simulink model "nfo"  (R2023b)
settings: Solver=FixedStepAuto  StartTime=0.0  StopTime=10.0  FixedStep=1e-4  RelTol=1e-3
values from neighbouring files (symbols this model uses):
  flux = 0.0059    [nfo.sldd]
  if_init = 40.0    [nfo.sldd]
  L = 8.5E-5    [nfo.sldd]
  Pn = 5.0    [nfo.sldd]
  Rs = 0.035    [nfo.sldd]
  Ts = 0.0001    [nfo.sldd]
  Udc = 24.0    [nfo.sldd]
undefined symbols (not defined in the file or in its folder): DiscIntNeverNeededParam, magnitude, PLL_I, PLL_P, sigbuilder_block
libraries: slpidlib x4, dspstat3 x1, mcbplantlib x1, autolibpmsmexterior x1
(part 1 of 2)
settings Model: DataDictionary=nfo.sldd  Creator=Administrator  LastModifiedBy=yanke
settings OptimizationCC: DefaultParameterBehavior=Inlined  UseDivisionForNetSlopeComputation=on  GainParamInheritBuiltInType=on  UseFloatMulNetSlope=on  InlineInvariantSignals=on  PassReuseOutputArgsAs=Individual arguments  ZeroExternalMemoryAtStartup=off  ZeroInternalMemoryAtStartup=off  NoFixptDivByZeroProtection=on  EfficientFloat2IntCast=on  LifeSpan=1  OptimizeBlockOrder=speed  DifferentSizesBufferReuse=on  EfficientTunableParamExpr=on
settings DebuggingCC: ParameterTunabilityLossMsg=error  UnconnectedInputMsg=warning  UnconnectedOutputMsg=warning  UnconnectedLineMsg=warning
settings HardwareCC: ProdBitPerPointer=32  ProdBitPerSizeT=32  ProdBitPerPtrDiffT=32  ProdLargestAtomicInteger=Long  ProdLargestAtomicFloat=Double  ProdWordSize=32  ProdLongLongMode=on  ProdHWDeviceType=ARM Compatible->ARM Cortex-M
settings ModelReferenceCC: EnableRefExpFcnMdlSchedulingChecks=on
settings SFSimCC: MATLABDynamicMemAlloc=off
settings RTWCC: Description=Embedded Coder  SystemTargetFile=ert.tlc  GenCodeOnly=on  TemplateMakefile=ert_default_tmf  GenerateReport=on  LaunchReport=on  GenerateCodeReplacementReport=on  DLArmComputeVersion=19.05
settings CodeAppCC: ForceParamTrailComments=on  IgnoreCustomStorageClasses=off  OperatorAnnotations=on  SimulinkDataObjDesc=on  SFDataObjDesc=on  CustomSymbolStrGlobalVar=rt$N$M  CustomSymbolStrType=$N$M  CustomSymbolStrFcn=$N$M$F  CustomSymbolStrMacro=$N$M  InsertBlockDesc=on
settings ERTTargetCC: TargetLangStandard=C99 (ISO)  CodeReplacementLibrary=ARM Cortex-M  GenerateSampleERTMain=on  IncludeMdlTerminateFcn=off  CombineSignalStateStructs=on  SupportComplex=off  SupportNonInlinedSFcns=on  InlinedParameterPlacement=NonHierarchical  ERTCustomFileTemplate=example_file_process.tlc  ERTFilePackagingFormat=CompactWithDataFile

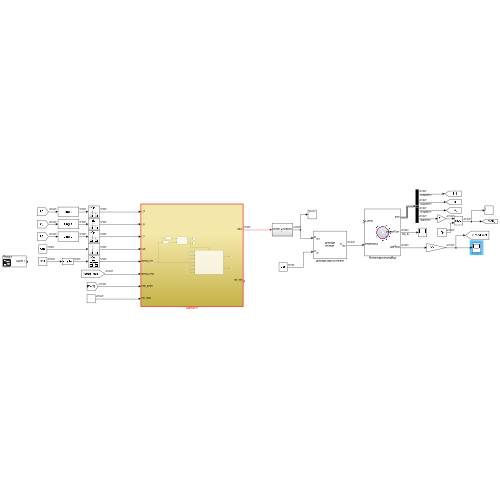
[thumbnail: Simulink's stored preview of the top-level diagram]
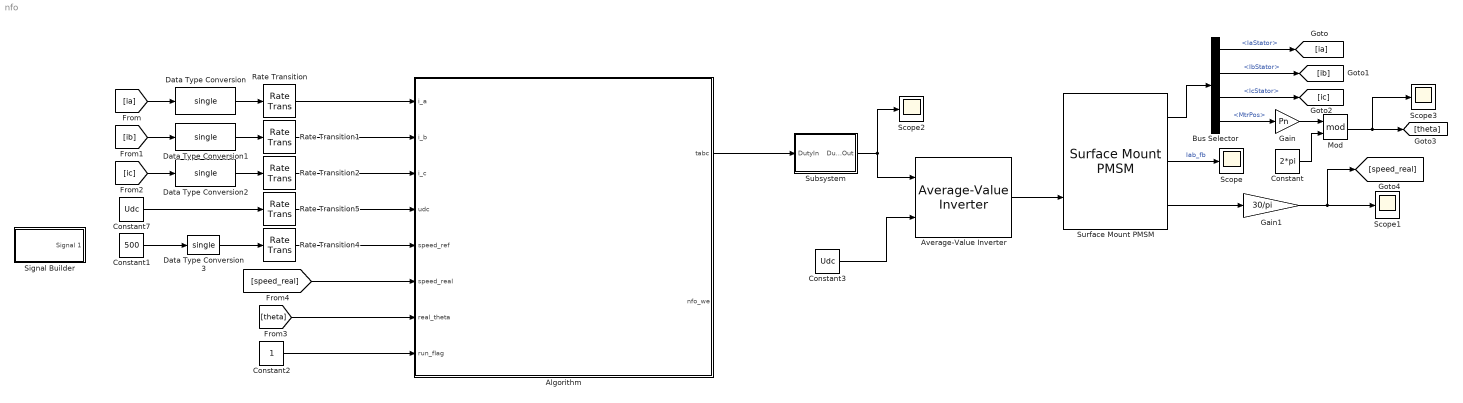
== system nfo ==
  Algorithm : Subsystem  TreatAsAtomicUnit=on
  Average-Value Inverter : mcbplantlib/Average-Value Inverter
  Bus Selector : BusSelector  OutputSignals=IaStator,IbStator,IcStator,MtrPos
  Constant : Constant  Value=2*pi
  Constant1 : Constant  Value=500
  Constant2 : Constant
  Constant3 : Constant  Value=Udc
  Constant7 : Constant  Value=Udc
  Data Type Conversion{,1..3} (4 alike) : DataTypeConversion  OutDataTypeStr=single  SaturateOnIntegerOverflow=off  RndMeth=Floor
  Gain : Gain  Gain=Pn
  Gain1 : Gain  Gain=30/pi
  Mod : Math  Operator=mod
  Rate Transition{,1..2,4..5} (5 alike) : RateTransition
  Scope{,1..3} (4 alike) : Scope
  Signal Builder : Subsystem  Tag=STV Subsys  LoadFcn=sigbuilder_block('load');  StartFcn=sigbuilder_block('start');  StopFcn=sigbuilder_block('stop');  ClipboardFcn=sigbuilder_block('clipboard');  mask(Sigbuilder block){tuvar=[0:10]}
      mask help: Simulink:masks:SigbuilderBlock_MD
      mask init:
      | if ~strcmp(get_param(bdroot(gcbh),'SimulationStatus'),'stopped') tuvar = sigbuilder_block('maskInit'); end
      settings: CopyFcn=sigbuilder_block('copy');  DeleteFcn=sigbuilder_block('delete');  ModelCloseFcn=sigbuilder_block('modelClose');  PreSaveFcn=sigbuilder_block('preSave');  PauseFcn=sigbuilder_block('pause');  ContinueFcn=sigbuilder_block('continue');  NameChangeFcn=sigbuilder_block('namechange');  OpenFcn=sigbuilder_block('open',[66 30 1269 684 ]);  CloseFcn=sigbuilder_block('close');
      mask Display: plot(0, 0, 100, 100,[2, 2, 32, 32, 2], [68, 8, 8, 68, 68],[32, 2], [38, 38], [32, 19, 2],[53, 60, 44], [32, 17, 17, 2],[16, 16, 31, 31]);txt = getActiveGroup(gcbh);text(2, 100, txt,'verticalAlignment', 'top');
  Subsystem : Subsystem
  Surface Mount PMSM : autolibpmsmexterior/Surface Mount PMSM  port_config=Torque  sim_type=Discrete  Ts=1e-4  P=Pn  Rs=Rs  Ldq_=L  KConstText=Permanent flux linkage constant (lambda_pm):  lambda_pm=flux  Ke=0.0059268  Kt=0.061  mechanical=[5.8e-5,0.0004924, 0]  idq0=[0 0]  theta_init=4/5  omega_init=0  KConst=flux  lambda_pm_calc=flux  RefBlkName='autolibpmsmexterior/Surface Mount PMSM'  aMode=5  Ldq="[0.0017      0.0017]"
  wires:
  Constant3/1 -> Average-Value Inverter/2
  Average-Value Inverter/1 -> Surface Mount PMSM/2
  Surface Mount PMSM/2 -> Scope/1  "Iab_fb"
  Surface Mount PMSM/1 -> Bus Selector/1
  Bus Selector/1 -> [ia]  "<IaStator>"
  Bus Selector/2 -> [ib]  "<IbStator>"
  Bus Selector/3 -> [ic]  "<IcStator>"
  Bus Selector/4 -> Gain/1  "<MtrPos>"
  Gain/1 -> Mod/1
  Constant/1 -> Mod/2
  Mod/1 -> Scope3/1, [theta]
  Data Type Conversion/1 -> Rate Transition/1
  [ia] -> Data Type Conversion/1
  [ib] -> Data Type Conversion1/1
  Data Type Conversion1/1 -> Rate Transition1/1
  Data Type Conversion2/1 -> Rate Transition2/1
  [ic] -> Data Type Conversion2/1
  Surface Mount PMSM/3 -> Gain1/1
  Gain1/1 -> [speed_real], Scope1/1
  Data Type Conversion3/1 -> Rate Transition4/1
  Subsystem/1(DutyOut) -> Average-Value Inverter/1, Scope2/1
  Algorithm/1(tabc) -> Subsystem/1(DutyIn)
  Rate Transition/1 -> Algorithm/1(i_a)
  Rate Transition1/1 -> Algorithm/2(i_b)
  Rate Transition2/1 -> Algorithm/3(i_c)
  Rate Transition5/1 -> Algorithm/4(udc)
  Constant7/1 -> Rate Transition5/1
  Rate Transition4/1 -> Algorithm/5(speed_ref)
  [speed_real] -> Algorithm/6(speed_real)
  [theta] -> Algorithm/7(real_theta)
  Constant2/1 -> Algorithm/8(run_flag)
  Constant1/1 -> Data Type Conversion3/1

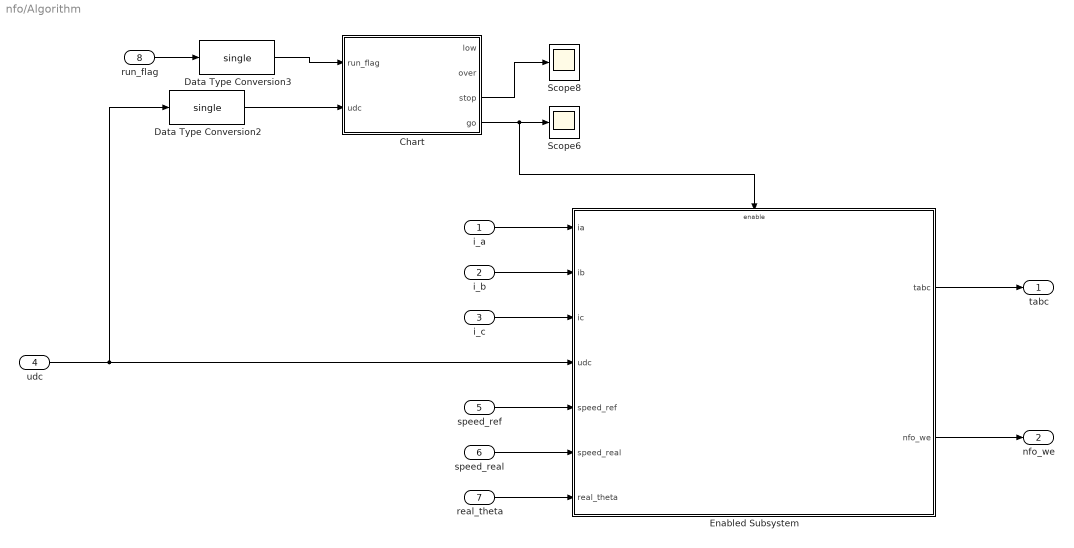
== system nfo/Algorithm ==
  i_a : Inport
  i_b : Inport  Port=2
  i_c : Inport  Port=3
  udc : Inport  Port=4
  speed_ref : Inport  Port=5
  speed_real : Inport  Port=6
  real_theta : Inport  Port=7
  run_flag : Inport  Port=8
  Chart : Stateflow chart  TreatAsAtomicUnit=on
  Data Type Conversion2 : DataTypeConversion  OutDataTypeStr=single  SaturateOnIntegerOverflow=off  RndMeth=Floor
  Data Type Conversion3 : DataTypeConversion  OutDataTypeStr=single  SaturateOnIntegerOverflow=off  RndMeth=Floor
  Enabled Subsystem : Subsystem  TreatAsAtomicUnit=on
  Scope6 : Scope
  Scope8 : Scope
  tabc : Outport
  nfo_we : Outport  Port=2
  wires:
  udc/1 -> Data Type Conversion2/1, Enabled Subsystem/4(udc)
  Data Type Conversion2/1 -> Chart/2(udc)
  run_flag/1 -> Data Type Conversion3/1
  Data Type Conversion3/1 -> Chart/1(run_flag)
  Chart/4(go) -> Enabled Subsystem/Enable, Scope6/1
  Chart/3(stop) -> Scope8/1
  i_a/1 -> Enabled Subsystem/1(ia)
  i_b/1 -> Enabled Subsystem/2(ib)
  i_c/1 -> Enabled Subsystem/3(ic)
  speed_ref/1 -> Enabled Subsystem/5(speed_ref)
  speed_real/1 -> Enabled Subsystem/6(speed_real)
  real_theta/1 -> Enabled Subsystem/7(real_theta)
  Enabled Subsystem/1(tabc) -> tabc/1
  Enabled Subsystem/2(nfo_we) -> nfo_we/1

== system nfo/Signal Builder ==
  Demux : Demux  Tag=STV Demux  Outputs=1
      settings: DisplayOption=none
  FromWs : FromWorkspace  Tag=STV FromWs  VariableName=tuvar
      SigBuilderData=|
      | common.afterFinalStr = 'Extrapolate'
      | common.sampleTime = 0
      | dataSet.timeRange = [0 10]
      | dataSet.name = 'Group 1'
      | sbobj.Groups.Name = 'Group 1'
      | sbobj.Groups.Signals.Name = 'Signal 1'
      | sbobj.Groups.Signals.XData = [0 4 4 7 7 10]
      | sbobj.Groups.Signals.YData = [302 302 700 700 -238 -238]
  Signal 1 : Outport  Tag=STV Outport
  wires:
  Demux/1 -> Signal 1/1
  FromWs/1 -> Demux/1

== system nfo/Subsystem ==
  DutyIn : Inport
  Constant : Constant  Value=0.5  SampleTime=-1
  Gain : Gain  Gain=1/8000  ParamDataTypeStr=single
  Gain1 : Gain  Gain=-1
  Sum : Sum  Inputs=|+-
  Sum1 : Sum  Inputs=|++
  DutyOut : Outport
  wires:
  Sum/1 -> Gain1/1
  Constant/1 -> Sum1/2, Sum/2
  DutyIn/1 -> Gain/1
  Gain1/1 -> Sum1/1
  Sum1/1 -> DutyOut/1
  Gain/1 -> Sum/1

== system nfo/Algorithm/Chart/low_vbus ==
  Input : Inport  OutDataTypeStr=single  PortDimensions=1
  f : TriggerPort  TriggerType=function-call  VariantControl=(inherit)
      settings: CopyFcn=Stateflow.SLINSF.SimulinkMan.removeBlockPreDeleteFcn  PreDeleteFcn=Stateflow.SLINSF.SimulinkMan.unsafePredeleteFcn
  Data Type Conversion : DataTypeConversion  OutDataTypeStr=boolean  SaturateOnIntegerOverflow=off  RndMeth=Floor
  Data Type Conversion1 : DataTypeConversion  OutDataTypeStr=single  SaturateOnIntegerOverflow=off  RndMeth=Floor
  NOR : Logic  Operator=NOT  IconShape=distinctive  OutDataTypeStr=boolean
  Relay : Relay  OnSwitchValue=20  OffSwitchValue=18
  out : Outport
  wires:
  Input/1 -> Relay/1
  Relay/1 -> Data Type Conversion/1
  Data Type Conversion/1 -> NOR/1
  NOR/1 -> Data Type Conversion1/1
  Data Type Conversion1/1 -> out/1

== system nfo/Algorithm/Chart/over_vbus ==
  Input : Inport  OutDataTypeStr=single  PortDimensions=1
  f : TriggerPort  TriggerType=function-call  VariantControl=(inherit)
      settings: CopyFcn=Stateflow.SLINSF.SimulinkMan.removeBlockPreDeleteFcn  PreDeleteFcn=Stateflow.SLINSF.SimulinkMan.unsafePredeleteFcn
  Relay : Relay  OnSwitchValue=28  OffSwitchValue=25
  out : Outport
  wires:
  Input/1 -> Relay/1
  Relay/1 -> out/1

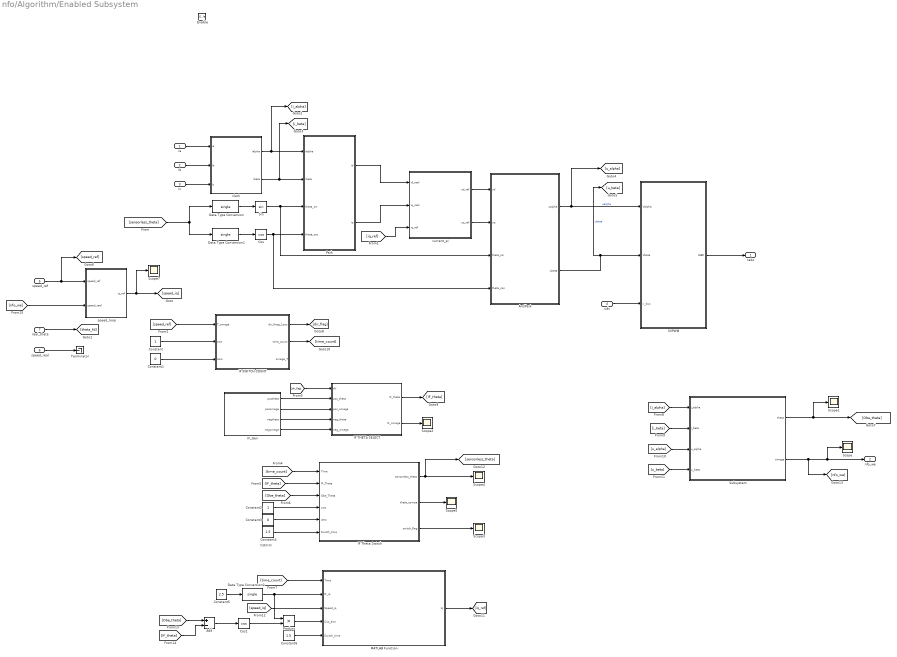
== system nfo/Algorithm/Enabled Subsystem ==
  note: 切换时间
  ia : Inport
  ib : Inport  Port=2
  ic : Inport  Port=3
  udc : Inport  Port=4
  speed_ref : Inport  Port=5
  speed_real : Inport  Port=6
  real_theta : Inport  Port=7
  Enable : EnablePort
  Add : Sum  Inputs=+-
  AntiPark : Subsystem
  Constant : Constant
  Constant1 : Constant  Value=0
  Constant2 : Constant  OutDataTypeStr=single
  Constant3 : Constant  Value=0  OutDataTypeStr=single
  Constant4 : Constant  Value=1.5  OutDataTypeStr=single
  Constant5 : Constant  Value=2.5
  Constant6 : Constant  Value=1.5
  Cos : Trigonometry  Operator=cos
  Cos1 : Trigonometry  Operator=cos
  Data Type Conversion : DataTypeConversion  OutDataTypeStr=single  SaturateOnIntegerOverflow=off  RndMeth=Floor
  Data Type Conversion1 : DataTypeConversion  OutDataTypeStr=single  SaturateOnIntegerOverflow=off  RndMeth=Floor
  Data Type Conversion2 : DataTypeConversion  OutDataTypeStr=single  SaturateOnIntegerOverflow=off  RndMeth=Floor
  IF SWITCH COUNT : MATLAB Function  TreatAsAtomicUnit=on
  IF THETA SELECT : MATLAB Function  TreatAsAtomicUnit=on
  "IF Theta Switch " : MATLAB Function  TreatAsAtomicUnit=on
  IF_Gen : Subsystem
  MATLAB Function : MATLAB Function  TreatAsAtomicUnit=on
  Park : Subsystem
  Product : Product
  SVPWM : Subsystem  TreatAsAtomicUnit=on
  Scope{,1..5,7} (7 alike) : Scope
  Sin : Trigonometry
  Subsystem : Subsystem
  Terminator : Terminator
  clark : Subsystem
  current_pi : Subsystem
  speed_loop : Subsystem
  tabc : Outport  OutputWhenDisabled=reset  InitialOutput=0
  nfo_we : Outport  Port=2
  wires:
  ic/1 -> clark/3(ic)
  AntiPark/2(ubeta) -> SVPWM/2(Vbeta), [u_beta]  "ubeta"
  IF_Gen/2(posomega) -> IF THETA SELECT/3(pos_omega)
  Data Type Conversion/1 -> Sin/1
  Park/1(id) -> current_pi/1(id_real)
  IF THETA SELECT/2(IF_omega) -> Scope2/1
  [i_alpha] -> Subsystem/1(i_alpha)
  ib/1 -> clark/2(ib)
  [speed_iq] -> MATLAB Function/3(Speed_iq)
  IF_Gen/1(postheta) -> IF THETA SELECT/2(pos_theta)
  Cos/1 -> AntiPark/4(theta_cos), Park/4(theta_cos)
  AntiPark/1(ualpha) -> [u_alpha], SVPWM/1(Valpha)  "ualpha"
  [time_count] -> MATLAB Function/1(Time)
  Subsystem/2(omega) -> [nfo_we], Scope/1, nfo_we/1
  Constant3/1 -> "IF Theta Switch "/5(zero)
  Sin/1 -> AntiPark/3(theta_sin), Park/3(theta_sin)
  IF SWITCH COUNT/1(dir_0neg_1pos) -> [dir_flag]
  "IF Theta Switch "/2(theta_compa) -> Scope5/1
  [i_beta] -> Subsystem/2(i_beta)
  Data Type Conversion1/1 -> Cos/1
  Constant6/1 -> MATLAB Function/5(Switch_time)
  Cos1/1 -> Product/2
  udc/1 -> SVPWM/3(v_bus)
  [sensorless_theta] -> Data Type Conversion/1, Data Type Conversion1/1
  [Obe_theta] -> Add/1
  [u_beta] -> Subsystem/4(u_beta)
  [iq_ref] -> current_pi/3(iq_ref)
  speed_ref/1 -> [speed_ref], speed_loop/1(speed_ref)
  clark/1(ialpha) -> [i_alpha], Park/1(ialpha)
  [u_alpha] -> Subsystem/3(u_alpha)
  IF_Gen/4(negomega) -> IF THETA SELECT/5(neg_omega)
  Subsystem/1(theta) -> Scope1/1, [Obe_theta]
  SVPWM/1(tABC) -> tabc/1
  ia/1 -> clark/1(ia)
  "IF Theta Switch "/1(sensorless_theta) -> Scope4/1, [sensorless_theta]
  real_theta/1 -> [theta_fd]
  [speed_ref] -> IF SWITCH COUNT/1(T_omega)
  Constant/1 -> IF SWITCH COUNT/2(one)
  [dir_flag] -> IF THETA SELECT/1(dir)
  current_pi/2(uq_ref) -> AntiPark/2(uq)
  Constant1/1 -> IF SWITCH COUNT/3(zero)
  clark/2(ibeta) -> [i_beta], Park/2(ibeta)
  [time_count] -> "IF Theta Switch "/1(Time)
  [Obe_theta] -> "IF Theta Switch "/3(Obe_Theta)
  Constant2/1 -> "IF Theta Switch "/4(one)
  [IF_theta] -> "IF Theta Switch "/2(IF_Theta)
  Park/2(iq) -> current_pi/2(iq_real)
  "IF Theta Switch "/3(switch_flag) -> Scope3/1
  Constant5/1 -> Data Type Conversion2/1
  IF THETA SELECT/1(IF_theta) -> [IF_theta]
  IF SWITCH COUNT/2(time_count) -> [time_count]
  IF_Gen/3(negtheta) -> IF THETA SELECT/4(neg_theta)
  Product/1 -> MATLAB Function/4(Cos_eror)
  Add/1 -> Cos1/1
  Constant4/1 -> "IF Theta Switch "/6(Switch_time)
  current_pi/1(ud_ref) -> AntiPark/1(ud)
  speed_loop/1(iq_ref) -> Scope7/1, [speed_iq]
  [IF_theta] -> Add/2
  MATLAB Function/1(Iq) -> [iq_ref]
  speed_real/1 -> Terminator/1
  [nfo_we] -> speed_loop/2(speed_real)
  Data Type Conversion2/1 -> Product/1, MATLAB Function/2(IF_iq)

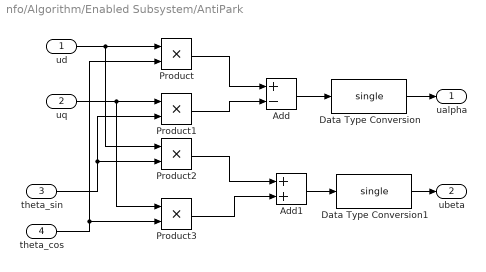
== system nfo/Algorithm/Enabled Subsystem/AntiPark ==
  ud : Inport
  uq : Inport  Port=2
  theta_sin : Inport  Port=3
  theta_cos : Inport  Port=4
  Add : Sum  Inputs=+-
  Add1 : Sum
  Data Type Conversion : DataTypeConversion  OutDataTypeStr=single  SaturateOnIntegerOverflow=off  RndMeth=Floor
  Data Type Conversion1 : DataTypeConversion  OutDataTypeStr=single  SaturateOnIntegerOverflow=off  RndMeth=Floor
  Product{,1..3} (4 alike) : Product
  ualpha : Outport  OutDataTypeStr=single
  ubeta : Outport  Port=2  OutDataTypeStr=single
  wires:
  Add1/1 -> Data Type Conversion1/1
  Product1/1 -> Add/2
  uq/1 -> Product3/1, Product1/1
  theta_cos/1 -> Product/2, Product3/2
  theta_sin/1 -> Product2/2, Product1/2
  ud/1 -> Product2/1, Product/1
  Product3/1 -> Add1/2
  Add/1 -> Data Type Conversion/1
  Product/1 -> Add/1
  Product2/1 -> Add1/1
  Data Type Conversion/1 -> ualpha/1
  Data Type Conversion1/1 -> ubeta/1

== system nfo/Algorithm/Enabled Subsystem/IF_Gen ==
  note: 对常数项积分，得到omega，在对omeg积分，得到theta
  IFneg : Subsystem  TreatAsAtomicUnit=on
      mask Display:
      | port_label('output',1,'negtheta','texmode','on');
      | port_label('output',2,'negomega','texmode','on');
      | 
      | fprintf('IFneg_theta');
  IFpos : Subsystem  TreatAsAtomicUnit=on
      mask Display:
      | port_label('output',1,'postheta','texmode','on');
      | port_label('output',2,'posomega','texmode','on');
      | 
      | fprintf('IFpos_theta');
  postheta : Outport
  posomega : Outport  Port=2
  negtheta : Outport  Port=3
  negomega : Outport  Port=4
  wires:
  IFpos/1(theta) -> postheta/1
  IFneg/2(omega) -> negomega/1
  IFneg/1(theta) -> negtheta/1
  IFpos/2(omega) -> posomega/1

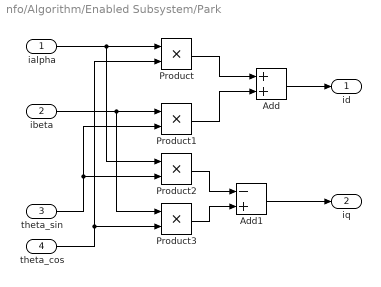
== system nfo/Algorithm/Enabled Subsystem/Park ==
  ialpha : Inport  OutDataTypeStr=single
  ibeta : Inport  Port=2  OutDataTypeStr=single
  theta_sin : Inport  Port=3  OutDataTypeStr=single
  theta_cos : Inport  Port=4  OutDataTypeStr=single
  Add : Sum  OutDataTypeStr=single  AccumDataTypeStr=single
  Add1 : Sum  Inputs=-+  OutDataTypeStr=single  AccumDataTypeStr=single
  Product{,1..3} (4 alike) : Product  OutDataTypeStr=single
  id : Outport  OutDataTypeStr=single
  iq : Outport  Port=2  OutDataTypeStr=single
  wires:
  theta_cos/1 -> Product/2, Product3/2
  ibeta/1 -> Product1/1, Product3/1
  Product1/1 -> Add/2
  Add1/1 -> iq/1
  Add/1 -> id/1
  Product3/1 -> Add1/2
  ialpha/1 -> Product/1, Product2/1
  Product2/1 -> Add1/1
  Product/1 -> Add/1
  theta_sin/1 -> Product1/2, Product2/2

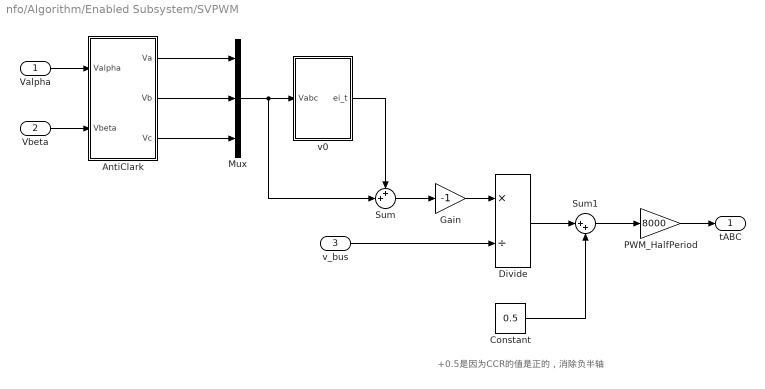
== system nfo/Algorithm/Enabled Subsystem/SVPWM ==
  note: +0.5是因为CCR的值是正的，消除负半轴
  Valpha : Inport  OutDataTypeStr=single
  Vbeta : Inport  Port=2  OutDataTypeStr=single
  v_bus : Inport  Port=3  OutDataTypeStr=single
  AntiClark : Subsystem
  Constant : Constant  Value=0.5  OutDataTypeStr=single
  Divide : Product  Inputs=*/  OutDataTypeStr=single
  Gain : Gain  Gain=-1  OutDataTypeStr=single
  Mux : Mux  Inputs=3
  PWM_HalfPeriod : Gain  Gain=8000  OutDataTypeStr=single
  Sum : Sum  Inputs=++|  OutDataTypeStr=single
  Sum1 : Sum  Inputs=|++  OutDataTypeStr=single
  v0 : Subsystem
  tABC : Outport  OutDataTypeStr=single
  wires:
  Valpha/1 -> AntiClark/1(Valpha)
  Vbeta/1 -> AntiClark/2(Vbeta)
  v0/1(ei_t) -> Sum/1
  AntiClark/1(Va) -> Mux/1
  AntiClark/2(Vb) -> Mux/2
  AntiClark/3(Vc) -> Mux/3
  Sum/1 -> Gain/1
  Mux/1 -> Sum/2, v0/1(Vabc)
  Divide/1 -> Sum1/1
  Constant/1 -> Sum1/2
  Sum1/1 -> PWM_HalfPeriod/1
  PWM_HalfPeriod/1 -> tABC/1
  v_bus/1 -> Divide/2
  Gain/1 -> Divide/1

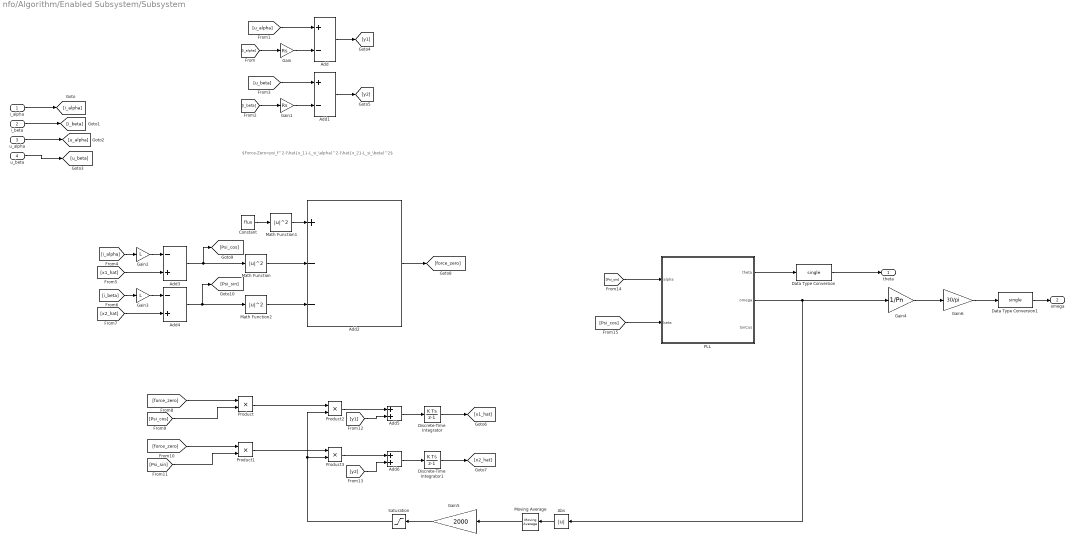
== system nfo/Algorithm/Enabled Subsystem/Subsystem ==
  note: $Force-Zero=psi_f^2-(\hat{x_1}-L_si_\alpha)^2-(\hat{x_2}-L_si_\beta)^2$
  i_alpha : Inport
  i_beta : Inport  Port=2
  u_alpha : Inport  Port=3
  u_beta : Inport  Port=4
  Abs : Abs  OutDataTypeStr=single  SaturateOnIntegerOverflow=off
  Add : Sum  Inputs=+-
  Add1 : Sum  Inputs=+-
  Add2 : Sum  Inputs=+--
  Add3 : Sum  Inputs=-+
  Add4 : Sum  Inputs=-+
  Add5 : Sum
  Add6 : Sum
  Constant : Constant  Value=flux
  Data Type Conversion : DataTypeConversion  OutDataTypeStr=single  SaturateOnIntegerOverflow=off  RndMeth=Floor
  Data Type Conversion1 : DataTypeConversion  OutDataTypeStr=single  SaturateOnIntegerOverflow=off  RndMeth=Floor
  Discrete-Time Integrator : DiscreteIntegrator  InitialCondition=0.011  SampleTime=-1  ICPrevOutput=DiscIntNeverNeededParam  ICPrevScaledInput=DiscIntNeverNeededParam
  Discrete-Time Integrator1 : DiscreteIntegrator  InitialCondition=-0.011  SampleTime=-1  ICPrevOutput=DiscIntNeverNeededParam  ICPrevScaledInput=DiscIntNeverNeededParam
  Gain : Gain  Gain=Rs
  Gain1 : Gain  Gain=Rs
  Gain2 : Gain  Gain=L
  Gain3 : Gain  Gain=L
  Gain4 : Gain  Gain=1/Pn
  Gain5 : Gain  Gain=2000  OutDataTypeStr=single
  Gain6 : Gain  Gain=30/pi
  Math Function : Math  Operator=magnitude^2
  Math Function1 : Math  Operator=magnitude^2
  Math Function2 : Math  Operator=magnitude^2
  Moving Average : dspstat3/Moving Average  Method=Exponential weighting  ForgettingFactorPort=off  SpecifyWindowLength=on  WindowLength=4  OverlapLength=3  AllowArbitraryInputLength=off  ForgettingFactor=0.99  SimulateUsing=Code generation
  PLL : Subsystem
  Product{,1..3} (4 alike) : Product
  Saturation : Saturate  UpperLimit=500e4  LowerLimit=100000  OutDataTypeStr=single
  theta : Outport
  omega : Outport  Port=2
  wires:
  i_alpha/1 -> [i_alpha]
  i_beta/1 -> [i_beta]
  [i_alpha] -> Gain/1
  Gain/1 -> Add/2
  u_alpha/1 -> [u_alpha]
  u_beta/1 -> [u_beta]
  [u_alpha] -> Add/1
  Gain1/1 -> Add1/2
  [i_beta] -> Gain1/1
  [u_beta] -> Add1/1
  Add/1 -> [y1]
  Add1/1 -> [y2]
  Constant/1 -> Math Function1/1
  [i_alpha] -> Gain2/1
  Gain2/1 -> Add3/1
  [x1_hat] -> Add3/2
  Add3/1 -> [Psi_cos], Math Function/1
  Math Function1/1 -> Add2/1
  Math Function/1 -> Add2/2
  [i_beta] -> Gain3/1
  [x2_hat] -> Add4/2
  Add4/1 -> [Psi_sin], Math Function2/1
  Gain3/1 -> Add4/1
  Math Function2/1 -> Add2/3
  Add2/1 -> [force_zero]
  [force_zero] -> Product/1
  [Psi_cos] -> Product/2
  [force_zero] -> Product1/1
  [Psi_sin] -> Product1/2
  Product1/1 -> Product3/1
  Product/1 -> Product2/1
  Product2/1 -> Add5/1
  [y1] -> Add5/2
  Product3/1 -> Add6/1
  [y2] -> Add6/2
  Add5/1 -> Discrete-Time Integrator/1
  Discrete-Time Integrator/1 -> [x1_hat]
  Add6/1 -> Discrete-Time Integrator1/1
  Discrete-Time Integrator1/1 -> [x2_hat]
  Abs/1 -> Moving Average/1
  Moving Average/1 -> Gain5/1
  Gain5/1 -> Saturation/1
  Saturation/1 -> Product2/2, Product3/2
  Gain4/1 -> Gain6/1
  Gain6/1 -> Data Type Conversion1/1
  Data Type Conversion1/1 -> omega/1
  Data Type Conversion/1 -> theta/1
  [Psi_sin] -> PLL/1(alpha)
  [Psi_cos] -> PLL/2(beta)
  PLL/1(theta) -> Data Type Conversion/1
  PLL/2(omega) -> Gain4/1, Abs/1

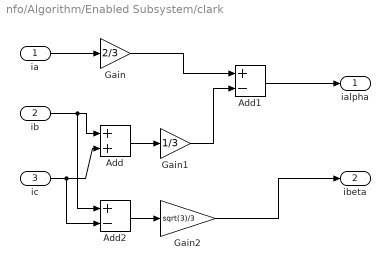
== system nfo/Algorithm/Enabled Subsystem/clark ==
  ia : Inport  OutDataTypeStr=single
  ib : Inport  Port=2  OutDataTypeStr=single
  ic : Inport  Port=3  OutDataTypeStr=single
  Add : Sum  OutDataTypeStr=single  AccumDataTypeStr=single
  Add1 : Sum  Inputs=+-  OutDataTypeStr=single  AccumDataTypeStr=single
  Add2 : Sum  Inputs=+-  OutDataTypeStr=single  AccumDataTypeStr=single
  Gain : Gain  Gain=2/3  ParamDataTypeStr=single
  Gain1 : Gain  Gain=1/3  ParamDataTypeStr=single
  Gain2 : Gain  Gain=sqrt(3)/3  ParamDataTypeStr=single
  ialpha : Outport  OutDataTypeStr=single
  ibeta : Outport  Port=2  OutDataTypeStr=single
  wires:
  ib/1 -> Add/1, Add2/1
  Gain1/1 -> Add1/2
  Add2/1 -> Gain2/1
  Add1/1 -> ialpha/1
  Gain/1 -> Add1/1
  ic/1 -> Add/2, Add2/2
  ia/1 -> Gain/1
  Add/1 -> Gain1/1
  Gain2/1 -> ibeta/1

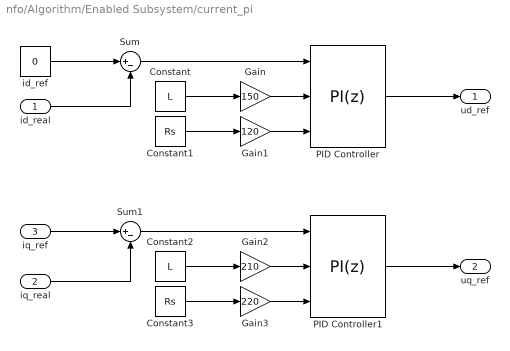
== system nfo/Algorithm/Enabled Subsystem/current_pi ==
  id_real : Inport
  iq_real : Inport  Port=2
  iq_ref : Inport  Port=3
  Constant : Constant  Value=L
  Constant1 : Constant  Value=Rs
  Constant2 : Constant  Value=L
  Constant3 : Constant  Value=Rs
  Gain : Gain  Gain=150
  Gain1 : Gain  Gain=120
  Gain2 : Gain  Gain=210
  Gain3 : Gain  Gain=220
  PID Controller : slpidlib/PID Controller  Controller=PI  Form=Parallel  TimeDomain=Discrete-time  UseExternalTs=off  SampleTime=-1  IntegratorMethod=Forward Euler  FilterMethod=Forward Euler  ControllerParametersSource=external  P=1  I=1  UseKiTs=off  D=0  N=100  UseFilter=on  TunerSelectOption=Transfer Function Based (PID Tuner App)  InitialConditionSource=internal  InitialConditionForIntegrator=0  InitialConditionForFilter=0  DifferentiatorICPrevScaledInput=0  ExternalReset=none  TrackingMode=off  Kt=1  LimitOutput=on  SatLimitsSource=internal  UpperSaturationLimit=Udc*0.9/sqrt(3)  LowerSaturationLimit=-Udc*0.9/sqrt(3)  LinearizeAsGain=on  AntiWindupMode=clamping  Kb=1  LimitIntegrator=off  UpperIntegratorSaturationLimit=inf  LowerIntegratorSaturationLimit=-inf  POutMin=[]  POutMax=[]  IOutMin=[]  IOutMax=[]  DOutMin=[]  DOutMax=[]  NOutMin=[]  NOutMax=[]  SumOutMin=[]  SumOutMax=[]  SaturationOutMin=[]  SaturationOutMax=[]  PParamMin=[]  PParamMax=[]  IParamMin=[]  IParamMax=[]  DParamMin=[]  DParamMax=[]  NParamMin=[]  NParamMax=[]  KbParamMin=[]  KbParamMax=[]  KtParamMin=[]  KtParamMax=[]  KbOutMin=[]  KbOutMax=[]  KtOutMin=[]  KtOutMax=[]  IntegratorOutMin=[]  IntegratorOutMax=[]  FilterOutMin=[]  FilterOutMax=[]  SumI1OutMin=[]  SumI1OutMax=[]  SumI2OutMin=[]  SumI2OutMax=[]  SumI3OutMin=[]  SumI3OutMax=[]  SumI4OutMin=[]  SumI4OutMax=[]  SumDOutMin=[]  SumDOutMax=[]  DifferentiatorOutMin=[]  DifferentiatorOutMax=[]  FilterDiffOutCoefMin=[]  FilterDiffOutCoefMax=[]  ReciprocalOutMin=[]  ReciprocalOutMax=[]  SumDenOutMin=[]  SumDenOutMax=[]  SumNumOutMin=[]  SumNumOutMax=[]  DivideOutMin=[]  DivideOutMax=[]  UdiffTsProdOutMin=[]  UdiffTsProdOutMax=[]  NTsProdOutMin=[]  NTsProdOutMax=[]  UintegralTsProdOutMin=[]  UintegralTsProdOutMax=[]  UngainTsProdOutMin=[]  UngainTsProdOutMax=[]  ClampingZeroOutDataTypeStr=Inherit: Inherit via back propagation  ClampingZeroOutMin=[]  ClampingZeroOutMax=[]  FilterDenConstantOutDataTypeStr=Inherit: Inherit via back propagation  FilterDenConstantOutMin=[]  FilterDenConstantOutMax=[]  PCopyOutDataTypeStr=Inherit: Inherit via back propagation  PCopyOutMin=[]  PCopyOutMax=[]  NCopyOutDataTypeStr=Inherit: Inherit via back propagation  NCopyOutMin=[]  NCopyOutMax=[]  IntegratorContinuousStateAttributes=''  IntegratorStateMustResolveToSignalObject=off  IntegratorRTWStateStorageClass=Auto  FilterContinuousStateAttributes=''  FilterStateMustResolveToSignalObject=off  FilterRTWStateStorageClass=Auto  ParallelPVariant=ExternalParameters  IdealPVariant=Disabled  IVariant=ExternalParameters  DVariant=Disabled  IntegratorVariant=Discrete  SatVariant=Enabled  AWVariant=DiscClampingParallel  PCopyVariant=Disabled  TRVariant=Disabled  FdbkBlocksVariant=Forward  IdealPFdbkVariant=Disabled  SatFdbkVariant=Disabled  DerivativeFilterVariant=Disabled  NVariant=Disabled  NCopyVariant=Disabled_SignalSpec  FilterICVariant=Disabled  IntegratorICVariant=InternalICs  ExternalResetVariant=Disabled  TRSumVariant=Passthrough  SumFdbkVariant=Disabled  SumVariant=Sum_PI  TsampFilterVariant=InternalTs  TsampNgainVariant=Passthrough  TsampIntegralVariant=Disabled_SignalSpec  ExternalSaturationOutDataTypeStr=Inherit: Same as second input
  PID Controller1 : slpidlib/PID Controller  Controller=PI  Form=Parallel  TimeDomain=Discrete-time  UseExternalTs=off  SampleTime=-1  IntegratorMethod=Forward Euler  FilterMethod=Forward Euler  ControllerParametersSource=external  P=1  I=1  UseKiTs=off  D=0  N=100  UseFilter=on  TunerSelectOption=Transfer Function Based (PID Tuner App)  InitialConditionSource=internal  InitialConditionForIntegrator=0  InitialConditionForFilter=0  DifferentiatorICPrevScaledInput=0  ExternalReset=none  TrackingMode=off  Kt=1  LimitOutput=on  SatLimitsSource=internal  UpperSaturationLimit=Udc*0.9/sqrt(3)  LowerSaturationLimit=-Udc*0.9/sqrt(3)  LinearizeAsGain=on  AntiWindupMode=clamping  Kb=1  LimitIntegrator=off  UpperIntegratorSaturationLimit=inf  LowerIntegratorSaturationLimit=-inf  POutMin=[]  POutMax=[]  IOutMin=[]  IOutMax=[]  DOutMin=[]  DOutMax=[]  NOutMin=[]  NOutMax=[]  SumOutMin=[]  SumOutMax=[]  SaturationOutMin=[]  SaturationOutMax=[]  PParamMin=[]  PParamMax=[]  IParamMin=[]  IParamMax=[]  DParamMin=[]  DParamMax=[]  NParamMin=[]  NParamMax=[]  KbParamMin=[]  KbParamMax=[]  KtParamMin=[]  KtParamMax=[]  KbOutMin=[]  KbOutMax=[]  KtOutMin=[]  KtOutMax=[]  IntegratorOutMin=[]  IntegratorOutMax=[]  FilterOutMin=[]  FilterOutMax=[]  SumI1OutMin=[]  SumI1OutMax=[]  SumI2OutMin=[]  SumI2OutMax=[]  SumI3OutMin=[]  SumI3OutMax=[]  SumI4OutMin=[]  SumI4OutMax=[]  SumDOutMin=[]  SumDOutMax=[]  DifferentiatorOutMin=[]  DifferentiatorOutMax=[]  FilterDiffOutCoefMin=[]  FilterDiffOutCoefMax=[]  ReciprocalOutMin=[]  ReciprocalOutMax=[]  SumDenOutMin=[]  SumDenOutMax=[]  SumNumOutMin=[]  SumNumOutMax=[]  DivideOutMin=[]  DivideOutMax=[]  UdiffTsProdOutMin=[]  UdiffTsProdOutMax=[]  NTsProdOutMin=[]  NTsProdOutMax=[]  UintegralTsProdOutMin=[]  UintegralTsProdOutMax=[]  UngainTsProdOutMin=[]  UngainTsProdOutMax=[]  ClampingZeroOutDataTypeStr=Inherit: Inherit via back propagation  ClampingZeroOutMin=[]  ClampingZeroOutMax=[]  FilterDenConstantOutDataTypeStr=Inherit: Inherit via back propagation  FilterDenConstantOutMin=[]  FilterDenConstantOutMax=[]  PCopyOutDataTypeStr=Inherit: Inherit via back propagation  PCopyOutMin=[]  PCopyOutMax=[]  NCopyOutDataTypeStr=Inherit: Inherit via back propagation  NCopyOutMin=[]  NCopyOutMax=[]  IntegratorContinuousStateAttributes=''  IntegratorStateMustResolveToSignalObject=off  IntegratorRTWStateStorageClass=Auto  FilterContinuousStateAttributes=''  FilterStateMustResolveToSignalObject=off  FilterRTWStateStorageClass=Auto  ParallelPVariant=ExternalParameters  IdealPVariant=Disabled  IVariant=ExternalParameters  DVariant=Disabled  IntegratorVariant=Discrete  SatVariant=Enabled  AWVariant=DiscClampingParallel  PCopyVariant=Disabled  TRVariant=Disabled  FdbkBlocksVariant=Forward  IdealPFdbkVariant=Disabled  SatFdbkVariant=Disabled  DerivativeFilterVariant=Disabled  NVariant=Disabled  NCopyVariant=Disabled_SignalSpec  FilterICVariant=Disabled  IntegratorICVariant=InternalICs  ExternalResetVariant=Disabled  TRSumVariant=Passthrough  SumFdbkVariant=Disabled  SumVariant=Sum_PI  TsampFilterVariant=InternalTs  TsampNgainVariant=Passthrough  TsampIntegralVariant=Disabled_SignalSpec  ExternalSaturationOutDataTypeStr=Inherit: Same as second input
  Sum : Sum  Inputs=|+-
  Sum1 : Sum  Inputs=|+-
  id_ref : Constant  Value=0
  ud_ref : Outport
  uq_ref : Outport  Port=2
  wires:
  id_ref/1 -> Sum/1
  id_real/1 -> Sum/2
  Sum/1 -> PID Controller/1
  PID Controller/1 -> ud_ref/1
  Gain/1 -> PID Controller/2
  Constant/1 -> Gain/1
  Gain1/1 -> PID Controller/3
  Constant1/1 -> Gain1/1
  Gain3/1 -> PID Controller1/3
  Constant2/1 -> Gain2/1
  Constant3/1 -> Gain3/1
  Gain2/1 -> PID Controller1/2
  Sum1/1 -> PID Controller1/1
  iq_ref/1 -> Sum1/1
  iq_real/1 -> Sum1/2
  PID Controller1/1 -> uq_ref/1

== system nfo/Algorithm/Enabled Subsystem/speed_loop ==
  note: 1.3 0.1
  speed_ref : Inport
  speed_real : Inport  Port=2
  PID Controller : slpidlib/PID Controller  Controller=PI  Form=Parallel  TimeDomain=Discrete-time  UseExternalTs=off  SampleTime=-1  IntegratorMethod=Forward Euler  FilterMethod=Forward Euler  ControllerParametersSource=internal  P=0.3  I=0.0003  UseKiTs=off  D=0  N=100  UseFilter=on  TunerSelectOption=Transfer Function Based (PID Tuner App)  InitialConditionSource=internal  InitialConditionForIntegrator=0  InitialConditionForFilter=0  DifferentiatorICPrevScaledInput=0  ExternalReset=none  TrackingMode=off  Kt=1  LimitOutput=on  SatLimitsSource=internal  UpperSaturationLimit=7  LowerSaturationLimit=-7  LinearizeAsGain=on  AntiWindupMode=clamping  Kb=1  LimitIntegrator=off  UpperIntegratorSaturationLimit=inf  LowerIntegratorSaturationLimit=-inf  POutMin=[]  POutMax=[]  IOutMin=[]  IOutMax=[]  DOutMin=[]  DOutMax=[]  NOutMin=[]  NOutMax=[]  SumOutMin=[]  SumOutMax=[]  SaturationOutMin=[]  SaturationOutMax=[]  PParamMin=[]  PParamMax=[]  IParamMin=[]  IParamMax=[]  DParamMin=[]  DParamMax=[]  NParamMin=[]  NParamMax=[]  KbParamMin=[]  KbParamMax=[]  KtParamMin=[]  KtParamMax=[]  KbOutMin=[]  KbOutMax=[]  KtOutMin=[]  KtOutMax=[]  IntegratorOutMin=[]  IntegratorOutMax=[]  FilterOutMin=[]  FilterOutMax=[]  SumI1OutMin=[]  SumI1OutMax=[]  SumI2OutMin=[]  SumI2OutMax=[]  SumI3OutMin=[]  SumI3OutMax=[]  SumI4OutMin=[]  SumI4OutMax=[]  SumDOutMin=[]  SumDOutMax=[]  DifferentiatorOutMin=[]  DifferentiatorOutMax=[]  FilterDiffOutCoefMin=[]  FilterDiffOutCoefMax=[]  ReciprocalOutMin=[]  ReciprocalOutMax=[]  SumDenOutMin=[]  SumDenOutMax=[]  SumNumOutMin=[]  SumNumOutMax=[]  DivideOutMin=[]  DivideOutMax=[]  UdiffTsProdOutMin=[]  UdiffTsProdOutMax=[]  NTsProdOutMin=[]  NTsProdOutMax=[]  UintegralTsProdOutMin=[]  UintegralTsProdOutMax=[]  UngainTsProdOutMin=[]  UngainTsProdOutMax=[]  ClampingZeroOutDataTypeStr=Inherit: Inherit via back propagation  ClampingZeroOutMin=[]  ClampingZeroOutMax=[]  FilterDenConstantOutDataTypeStr=Inherit: Inherit via back propagation  FilterDenConstantOutMin=[]  FilterDenConstantOutMax=[]  PCopyOutDataTypeStr=Inherit: Inherit via back propagation  PCopyOutMin=[]  PCopyOutMax=[]  NCopyOutDataTypeStr=Inherit: Inherit via back propagation  NCopyOutMin=[]  NCopyOutMax=[]  IntegratorContinuousStateAttributes=''  IntegratorStateMustResolveToSignalObject=off  IntegratorRTWStateStorageClass=Auto  FilterContinuousStateAttributes=''  FilterStateMustResolveToSignalObject=off  FilterRTWStateStorageClass=Auto  ParallelPVariant=InternalParameters  IdealPVariant=Disabled  IVariant=InternalParameters  DVariant=Disabled  IntegratorVariant=Discrete  SatVariant=Enabled  AWVariant=DiscClampingParallel  PCopyVariant=Disabled  TRVariant=Disabled  FdbkBlocksVariant=Forward  IdealPFdbkVariant=Disabled  SatFdbkVariant=Disabled  DerivativeFilterVariant=Disabled  NVariant=Disabled  NCopyVariant=Disabled_SignalSpec  FilterICVariant=Disabled  IntegratorICVariant=InternalICs  ExternalResetVariant=Disabled  TRSumVariant=Passthrough  SumFdbkVariant=Disabled  SumVariant=Sum_PI  TsampFilterVariant=InternalTs  TsampNgainVariant=Passthrough  TsampIntegralVariant=Disabled_SignalSpec  ExternalSaturationOutDataTypeStr=Inherit: Same as second input
  Sum : Sum  Inputs=|+-
  iq_ref : Outport
  wires:
  speed_ref/1 -> Sum/1
  speed_real/1 -> Sum/2
  Sum/1 -> PID Controller/1
  PID Controller/1 -> iq_ref/1

== system nfo/Algorithm/Enabled Subsystem/IF_Gen/IFneg ==
  Constant : Constant  Value=if_init  OutDataTypeStr=single
  Discrete-Time Integrator : DiscreteIntegrator  SampleTime=-1  ICPrevOutput=DiscIntNeverNeededParam  ICPrevScaledInput=DiscIntNeverNeededParam
  Gain : Gain  Gain=-1
  integrator : Subsystem
  theta : Outport  OutDataTypeStr=single
  omega : Outport  Port=2  OutDataTypeStr=single
  wires:
  integrator/1(y(k-1)) -> theta/1
  Constant/1 -> Gain/1
  Gain/1 -> Discrete-Time Integrator/1
  Discrete-Time Integrator/1 -> omega/1, integrator/1(x(k))

== system nfo/Algorithm/Enabled Subsystem/IF_Gen/IFpos ==
  Constant : Constant  Value=if_init  OutDataTypeStr=single
  Discrete-Time Integrator : DiscreteIntegrator  SampleTime=-1  ICPrevOutput=DiscIntNeverNeededParam  ICPrevScaledInput=DiscIntNeverNeededParam
  Scope : Scope
  Scope1 : Scope
  integrator : Subsystem
  theta : Outport  OutDataTypeStr=single
  omega : Outport  Port=2  OutDataTypeStr=single
  wires:
  integrator/1(y(k-1)) -> Scope1/1, theta/1
  Constant/1 -> Discrete-Time Integrator/1
  Discrete-Time Integrator/1 -> Scope/1, omega/1, integrator/1(x(k))

== system nfo/Algorithm/Enabled Subsystem/SVPWM/AntiClark ==
  Valpha : Inport  OutDataTypeStr=single
  Vbeta : Inport  Port=2  OutDataTypeStr=single
  Gain : Gain  Gain=-1/2  OutDataTypeStr=single
  Gain1 : Gain  Gain=sqrt(3)/2  OutDataTypeStr=single
  Sum : Sum  Inputs=|++  OutDataTypeStr=single
  Sum1 : Sum  Inputs=-+|  OutDataTypeStr=single
  Va : Outport  OutDataTypeStr=single
  Vb : Outport  Port=2  OutDataTypeStr=single
  Vc : Outport  Port=3  OutDataTypeStr=single
  wires:
  Valpha/1 -> Gain/1, Va/1
  Vbeta/1 -> Gain1/1
  Gain/1 -> Sum1/2, Sum/1
  Sum/1 -> Vb/1
  Gain1/1 -> Sum/2, Sum1/1
  Sum1/1 -> Vc/1

== system nfo/Algorithm/Enabled Subsystem/SVPWM/v0 ==
  Vabc : Inport  OutDataTypeStr=single
  Demux : Demux  Outputs=3
  Gain : Gain  Gain=-1/2  OutDataTypeStr=single
  Min : MinMax  Inputs=3  OutDataTypeStr=single
  Min1 : MinMax  Function=max  Inputs=3  OutDataTypeStr=single
  Sum : Sum  Inputs=|++  OutDataTypeStr=single
  ei_t : Outport  OutDataTypeStr=single
  wires:
  Min/1 -> Sum/1
  Sum/1 -> Gain/1
  Min1/1 -> Sum/2
  Gain/1 -> ei_t/1
  Vabc/1 -> Demux/1
  Demux/1 -> Min1/1, Min/1
  Demux/2 -> Min/2, Min1/2
  Demux/3 -> Min1/3, Min/3

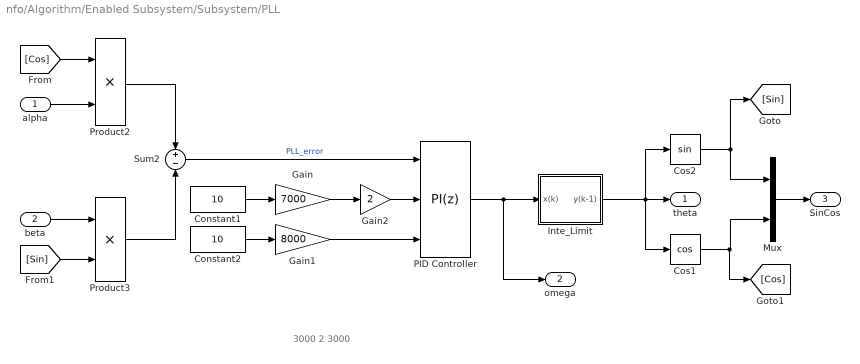
== system nfo/Algorithm/Enabled Subsystem/Subsystem/PLL ==
  note: 3000 2 3000
  alpha : Inport  OutDataTypeStr=single
  beta : Inport  Port=2  OutDataTypeStr=single
  Constant1 : Constant  Value=10  OutDataTypeStr=single
  Constant2 : Constant  Value=10  OutDataTypeStr=single
  Cos1 : Trigonometry  Operator=cos
  Cos2 : Trigonometry
  Gain : Gain  Gain=7000
  Gain1 : Gain  Gain=8000
  Gain2 : Gain  Gain=2
  Inte_Limit : Subsystem
  Mux : Mux  Inputs=2
  PID Controller : slpidlib/PID Controller  Controller=PI  Form=Parallel  TimeDomain=Discrete-time  UseExternalTs=off  SampleTime=-1  IntegratorMethod=Forward Euler  FilterMethod=Forward Euler  ControllerParametersSource=external  P=2*PLL_P*PLL_I  I=PLL_I*PLL_I  UseKiTs=off  D=0  N=100  UseFilter=on  TunerSelectOption=Transfer Function Based (PID Tuner App)  ZeroCross=off  InitialConditionSource=internal  InitialConditionForIntegrator=0  InitialConditionForFilter=0  DifferentiatorICPrevScaledInput=0  ExternalReset=none  TrackingMode=off  Kt=1  LimitOutput=on  SatLimitsSource=internal  UpperSaturationLimit=2500  LowerSaturationLimit=-2500  LinearizeAsGain=on  AntiWindupMode=none  Kb=1  LimitIntegrator=off  UpperIntegratorSaturationLimit=inf  LowerIntegratorSaturationLimit=-inf  POutMin=[]  POutMax=[]  IOutMin=[]  IOutMax=[]  DOutMin=[]  DOutMax=[]  NOutMin=[]  NOutMax=[]  SumOutMin=[]  SumOutMax=[]  SaturationOutMin=[]  SaturationOutMax=[]  PParamMin=[]  PParamMax=[]  IParamMin=[]  IParamMax=[]  DParamMin=[]  DParamMax=[]  NParamMin=[]  NParamMax=[]  KbParamMin=[]  KbParamMax=[]  KtParamMin=[]  KtParamMax=[]  KbOutMin=[]  KbOutMax=[]  KtOutMin=[]  KtOutMax=[]  IntegratorOutMin=[]  IntegratorOutMax=[]  FilterOutMin=[]  FilterOutMax=[]  SumI1OutMin=[]  SumI1OutMax=[]  SumI2OutMin=[]  SumI2OutMax=[]  SumI3OutMin=[]  SumI3OutMax=[]  SumI4OutMin=[]  SumI4OutMax=[]  SumDOutMin=[]  SumDOutMax=[]  DifferentiatorOutMin=[]  DifferentiatorOutMax=[]  FilterDiffOutCoefMin=[]  FilterDiffOutCoefMax=[]  ReciprocalOutMin=[]  ReciprocalOutMax=[]  SumDenOutMin=[]  SumDenOutMax=[]  SumNumOutMin=[]  SumNumOutMax=[]  DivideOutMin=[]  DivideOutMax=[]  UdiffTsProdOutMin=[]  UdiffTsProdOutMax=[]  NTsProdOutMin=[]  NTsProdOutMax=[]  UintegralTsProdOutMin=[]  UintegralTsProdOutMax=[]  UngainTsProdOutMin=[]  UngainTsProdOutMax=[]  ClampingZeroOutDataTypeStr=Inherit: Inherit via back propagation  ClampingZeroOutMin=[]  ClampingZeroOutMax=[]  FilterDenConstantOutDataTypeStr=Inherit: Inherit via back propagation  FilterDenConstantOutMin=[]  FilterDenConstantOutMax=[]  PCopyOutDataTypeStr=Inherit: Inherit via back propagation  PCopyOutMin=[]  PCopyOutMax=[]  NCopyOutDataTypeStr=Inherit: Inherit via back propagation  NCopyOutMin=[]  NCopyOutMax=[]  IntegratorContinuousStateAttributes=''  IntegratorStateMustResolveToSignalObject=off  IntegratorRTWStateStorageClass=Auto  FilterContinuousStateAttributes=''  FilterStateMustResolveToSignalObject=off  FilterRTWStateStorageClass=Auto  ParallelPVariant=ExternalParameters  IdealPVariant=Disabled  IVariant=ExternalParameters  DVariant=Disabled  IntegratorVariant=Discrete  SatVariant=Enabled  AWVariant=Passthrough  PCopyVariant=Disabled  TRVariant=Disabled  FdbkBlocksVariant=Forward  IdealPFdbkVariant=Disabled  SatFdbkVariant=Disabled  DerivativeFilterVariant=Disabled  NVariant=Disabled  NCopyVariant=Disabled_SignalSpec  FilterICVariant=Disabled  IntegratorICVariant=InternalICs  ExternalResetVariant=Disabled  TRSumVariant=Passthrough  SumFdbkVariant=Disabled  SumVariant=Sum_PI  TsampFilterVariant=InternalTs  TsampNgainVariant=Passthrough  TsampIntegralVariant=Disabled_SignalSpec  ExternalSaturationOutDataTypeStr=Inherit: Same as second input
  Product2 : Product  OutDataTypeStr=single
  Product3 : Product  OutDataTypeStr=single
  Sum2 : Sum  Inputs=+|-  OutDataTypeStr=single
  theta : Outport  OutDataTypeStr=single
  omega : Outport  Port=2  OutDataTypeStr=single
  SinCos : Outport  Port=3  OutDataTypeStr=single
  wires:
  Product2/1 -> Sum2/1
  Inte_Limit/1(y(k-1)) -> Cos2/1, Cos1/1, theta/1
  Product3/1 -> Sum2/2
  alpha/1 -> Product2/2
  beta/1 -> Product3/1
  Sum2/1 -> PID Controller/1  "PLL_error"
  Constant1/1 -> Gain/1
  Gain/1 -> Gain2/1
  Constant2/1 -> Gain1/1
  Gain1/1 -> PID Controller/3
  Mux/1 -> SinCos/1
  Cos2/1 -> Mux/1, [Sin]
  Cos1/1 -> [Cos], Mux/2
  [Cos] -> Product2/1
  [Sin] -> Product3/2
  Gain2/1 -> PID Controller/2
  PID Controller/1 -> omega/1, Inte_Limit/1(x(k))

== system nfo/Algorithm/Enabled Subsystem/IF_Gen/IFneg/integrator ==
  note: $y(k)=x(k)*T_s+y(k-1)$
  x(k) : Inport  OutDataTypeStr=single
  RangeLimit : Subsystem
  Sum1 : Sum  Inputs=|++  OutDataTypeStr=single
  Ts : Gain  Gain=Ts  OutDataTypeStr=single
  Unit Delay : UnitDelay  SampleTime=-1  HasFrameUpgradeWarning=on
  y(k-1) : Outport  OutDataTypeStr=single
  wires:
  RangeLimit/1(Theta) -> Unit Delay/1
  Unit Delay/1 -> Sum1/2, y(k-1)/1
  Sum1/1 -> RangeLimit/1(In)  "y(k)"
  Ts/1 -> Sum1/1
  x(k)/1 -> Ts/1

== system nfo/Algorithm/Enabled Subsystem/IF_Gen/IFpos/integrator ==
  note: $y(k)=x(k)*T_s+y(k-1)$
  x(k) : Inport  OutDataTypeStr=single
  RangeLimit : Subsystem
  Sum1 : Sum  Inputs=|++  OutDataTypeStr=single
  Ts : Gain  Gain=Ts  OutDataTypeStr=single
  Unit Delay : UnitDelay  SampleTime=-1  HasFrameUpgradeWarning=on
  y(k-1) : Outport  OutDataTypeStr=single
  wires:
  x(k)/1 -> Ts/1
  Ts/1 -> Sum1/1
  Sum1/1 -> RangeLimit/1(In)  "y(k)"
  Unit Delay/1 -> y(k-1)/1, Sum1/2
  RangeLimit/1(Theta) -> Unit Delay/1

== system nfo/Algorithm/Enabled Subsystem/Subsystem/PLL/Inte_Limit ==
  x(k) : Inport  OutDataTypeStr=single
  Delay : Delay  DelayLength=1
  Sum1 : Sum  Inputs=|++  OutDataTypeStr=single
  Ts : Gain  Gain=Ts  OutDataTypeStr=single
  xianfu : Subsystem
  y(k-1) : Outport  OutDataTypeStr=single
  wires:
  x(k)/1 -> Ts/1
  Ts/1 -> Sum1/1
  Sum1/1 -> xianfu/1(In)
  Delay/1 -> y(k-1)/1, Sum1/2
  xianfu/1(Theta) -> Delay/1

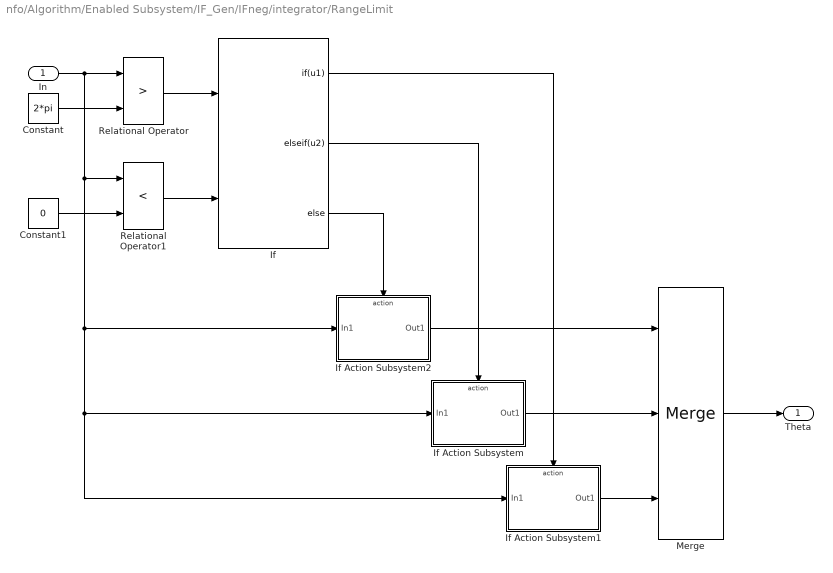
== system nfo/Algorithm/Enabled Subsystem/IF_Gen/IFneg/integrator/RangeLimit ==
  In : Inport  OutDataTypeStr=single
  Constant : Constant  Value=2*pi  OutDataTypeStr=single  SampleTime=-1
  Constant1 : Constant  Value=0  OutDataTypeStr=single  SampleTime=-1
  If : If  NumInputs=2  IfExpression=u1  ElseIfExpressions=u2
  If Action Subsystem : Subsystem  TreatAsAtomicUnit=on
  If Action Subsystem1 : Subsystem  TreatAsAtomicUnit=on
  If Action Subsystem2 : Subsystem  TreatAsAtomicUnit=on
  Merge : Merge  Inputs=3
  Relational Operator : RelationalOperator  Operator=>  OutDataTypeStr=boolean  RndMeth=Simplest  InputSameDT=off
  Relational Operator1 : RelationalOperator  Operator=<  OutDataTypeStr=boolean  RndMeth=Simplest  InputSameDT=off
  Theta : Outport  OutDataTypeStr=single
  wires:
  If Action Subsystem1/1(Out1) -> Merge/3
  If Action Subsystem/1(Out1) -> Merge/2
  If Action Subsystem2/1(Out1) -> Merge/1
  If/1 -> If Action Subsystem1/Action
  If/2 -> If Action Subsystem/Action
  If/3 -> If Action Subsystem2/Action
  Merge/1 -> Theta/1
  Relational Operator1/1 -> If/2
  In/1 -> Relational Operator/1, If Action Subsystem/1(In1), If Action Subsystem1/1(In1), If Action Subsystem2/1(In1), Relational Operator1/1
  Constant1/1 -> Relational Operator1/2
  Constant/1 -> Relational Operator/2
  Relational Operator/1 -> If/1

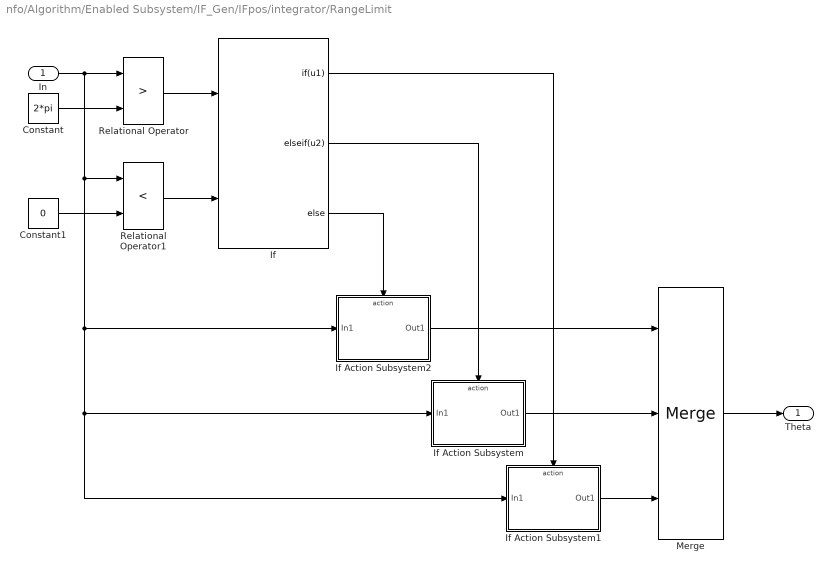
== system nfo/Algorithm/Enabled Subsystem/IF_Gen/IFpos/integrator/RangeLimit ==
  In : Inport  OutDataTypeStr=single
  Constant : Constant  Value=2*pi  OutDataTypeStr=single  SampleTime=-1
  Constant1 : Constant  Value=0  OutDataTypeStr=single  SampleTime=-1
  If : If  NumInputs=2  IfExpression=u1  ElseIfExpressions=u2
  If Action Subsystem : Subsystem  TreatAsAtomicUnit=on
  If Action Subsystem1 : Subsystem  TreatAsAtomicUnit=on
  If Action Subsystem2 : Subsystem  TreatAsAtomicUnit=on
  Merge : Merge  Inputs=3
  Relational Operator : RelationalOperator  Operator=>  OutDataTypeStr=boolean  RndMeth=Simplest  InputSameDT=off
  Relational Operator1 : RelationalOperator  Operator=<  OutDataTypeStr=boolean  RndMeth=Simplest  InputSameDT=off
  Theta : Outport  OutDataTypeStr=single
  wires:
  Relational Operator/1 -> If/1
  Constant/1 -> Relational Operator/2
  Constant1/1 -> Relational Operator1/2
  In/1 -> Relational Operator1/1, If Action Subsystem2/1(In1), If Action Subsystem1/1(In1), If Action Subsystem/1(In1), Relational Operator/1
  Relational Operator1/1 -> If/2
  Merge/1 -> Theta/1
  If/3 -> If Action Subsystem2/Action
  If/2 -> If Action Subsystem/Action
  If/1 -> If Action Subsystem1/Action
  If Action Subsystem2/1(Out1) -> Merge/1
  If Action Subsystem/1(Out1) -> Merge/2
  If Action Subsystem1/1(Out1) -> Merge/3

== system nfo/Algorithm/Enabled Subsystem/Subsystem/PLL/Inte_Limit/xianfu ==
  In : Inport  OutDataTypeStr=single
  Constant : Constant  Value=2*pi  OutDataTypeStr=single  SampleTime=-1
  Constant1 : Constant  Value=0  OutDataTypeStr=single  SampleTime=-1
  If : If  NumInputs=2  IfExpression=u1  ElseIfExpressions=u2
  If Action Subsystem : Subsystem  TreatAsAtomicUnit=on
  If Action Subsystem1 : Subsystem  TreatAsAtomicUnit=on
  If Action Subsystem2 : Subsystem  TreatAsAtomicUnit=on
  Merge : Merge  Inputs=3
  Relational Operator : RelationalOperator  Operator=>  OutDataTypeStr=boolean  RndMeth=Simplest  InputSameDT=off
  Relational Operator1 : RelationalOperator  Operator=<  OutDataTypeStr=boolean  RndMeth=Simplest  InputSameDT=off
  Theta : Outport  OutDataTypeStr=single
  wires:
  Relational Operator/1 -> If/1
  Constant/1 -> Relational Operator/2
  Constant1/1 -> Relational Operator1/2
  In/1 -> Relational Operator1/1, If Action Subsystem2/1(In1), If Action Subsystem1/1(In1), If Action Subsystem/1(In1), Relational Operator/1
  Relational Operator1/1 -> If/2
  Merge/1 -> Theta/1
  If/3 -> If Action Subsystem2/Action
  If/2 -> If Action Subsystem/Action
  If/1 -> If Action Subsystem1/Action
  If Action Subsystem2/1(Out1) -> Merge/1
  If Action Subsystem/1(Out1) -> Merge/2
  If Action Subsystem1/1(Out1) -> Merge/3

== system nfo/Algorithm/Enabled Subsystem/IF_Gen/IFneg/integrator/RangeLimit/If Action Subsystem ==
  In1 : Inport  OutDataTypeStr=single
  Action Port : ActionPort  ActionPortLabel=elseif(u2)
  Constant : Constant  Value=2*pi  OutDataTypeStr=single  SampleTime=-1
  Sum : Sum  Inputs=|++  OutDataTypeStr=single
  Out1 : Outport  OutDataTypeStr=single
  wires:
  Sum/1 -> Out1/1
  Constant/1 -> Sum/2
  In1/1 -> Sum/1

== system nfo/Algorithm/Enabled Subsystem/IF_Gen/IFneg/integrator/RangeLimit/If Action Subsystem1 ==
  In1 : Inport  OutDataTypeStr=single
  Action Port : ActionPort  ActionPortLabel=if(u1)
  Constant : Constant  Value=2*pi  OutDataTypeStr=single  SampleTime=-1
  Sum : Sum  Inputs=|+-  OutDataTypeStr=single
  Out1 : Outport  OutDataTypeStr=single
  wires:
  Sum/1 -> Out1/1
  Constant/1 -> Sum/2
  In1/1 -> Sum/1

== system nfo/Algorithm/Enabled Subsystem/IF_Gen/IFneg/integrator/RangeLimit/If Action Subsystem2 ==
  In1 : Inport  OutDataTypeStr=single
  Action Port : ActionPort  ActionPortLabel=else
  Out1 : Outport  OutDataTypeStr=single
  wires:
  In1/1 -> Out1/1

== system nfo/Algorithm/Enabled Subsystem/IF_Gen/IFpos/integrator/RangeLimit/If Action Subsystem ==
  In1 : Inport  OutDataTypeStr=single
  Action Port : ActionPort  ActionPortLabel=elseif(u2)
  Constant : Constant  Value=2*pi  OutDataTypeStr=single  SampleTime=-1
  Sum : Sum  Inputs=|++  OutDataTypeStr=single
  Out1 : Outport  OutDataTypeStr=single
  wires:
  In1/1 -> Sum/1
  Constant/1 -> Sum/2
  Sum/1 -> Out1/1

== system nfo/Algorithm/Enabled Subsystem/IF_Gen/IFpos/integrator/RangeLimit/If Action Subsystem1 ==
  In1 : Inport  OutDataTypeStr=single
  Action Port : ActionPort  ActionPortLabel=if(u1)
  Constant : Constant  Value=2*pi  OutDataTypeStr=single  SampleTime=-1
  Sum : Sum  Inputs=|+-  OutDataTypeStr=single
  Out1 : Outport  OutDataTypeStr=single
  wires:
  In1/1 -> Sum/1
  Constant/1 -> Sum/2
  Sum/1 -> Out1/1

== system nfo/Algorithm/Enabled Subsystem/IF_Gen/IFpos/integrator/RangeLimit/If Action Subsystem2 ==
  In1 : Inport  OutDataTypeStr=single
  Action Port : ActionPort  ActionPortLabel=else
  Out1 : Outport  OutDataTypeStr=single
  wires:
  In1/1 -> Out1/1

== system nfo/Algorithm/Enabled Subsystem/Subsystem/PLL/Inte_Limit/xianfu/If Action Subsystem ==
  In1 : Inport  OutDataTypeStr=single
  Action Port : ActionPort  ActionPortLabel=elseif(u2)
  Constant : Constant  Value=2*pi  OutDataTypeStr=single  SampleTime=-1
  Sum : Sum  Inputs=|++  OutDataTypeStr=single
  Out1 : Outport  OutDataTypeStr=single
  wires:
  In1/1 -> Sum/1
  Constant/1 -> Sum/2
  Sum/1 -> Out1/1

== system nfo/Algorithm/Enabled Subsystem/Subsystem/PLL/Inte_Limit/xianfu/If Action Subsystem1 ==
  In1 : Inport  OutDataTypeStr=single
  Action Port : ActionPort  ActionPortLabel=if(u1)
  Constant : Constant  Value=2*pi  OutDataTypeStr=single  SampleTime=-1
  Sum : Sum  Inputs=|+-  OutDataTypeStr=single
  Out1 : Outport  OutDataTypeStr=single
  wires:
  In1/1 -> Sum/1
  Constant/1 -> Sum/2
  Sum/1 -> Out1/1

== system nfo/Algorithm/Enabled Subsystem/Subsystem/PLL/Inte_Limit/xianfu/If Action Subsystem2 ==
  In1 : Inport  OutDataTypeStr=single
  Action Port : ActionPort  ActionPortLabel=else
  Out1 : Outport  OutDataTypeStr=single
  wires:
  In1/1 -> Out1/1

== matlab function nfo/Algorithm/Enabled Subsystem/IF THETA SELECT ==
  data: dir input; IF_theta output; pos_theta input; pos_omega input; neg_theta input; neg_omega input; IF_omega output
function [IF_theta, IF_omega]= fcn(dir,pos_theta,pos_omega,neg_theta,neg_omega)

if dir == 0
    IF_theta  = neg_theta;
    IF_omega = neg_omega;
else
    IF_theta = pos_theta;
    IF_omega = pos_omega;
end

== matlab function nfo/Algorithm/Enabled Subsystem/IF SWITCH COUNT ==
  data: T_omega input; dir_0neg_1pos output; one input; zero input; time_count output; omega_T output
function [dir_0neg_1pos,time_count,omega_T]= fcn(T_omega,one,zero)

%这个函数就是一个计数器，并且设置转动方向

time_count=zero; %一直增加的计数值
dir_0neg_1pos = zero; %设置方向
omega_T = T_omega; %给定角速度

%定义持久变量
persistent time
if isempty(time)
    time=0;
end


if(T_omega>30)
    %正转
    dir_0neg_1pos = one; % one就是1 zero就是0
    time = time + 0.0001; %运行频率为10Khz
    time_count = time;
elseif(T_omega<-30)
    %反转
    dir_0neg_1pos = zero; 
    time = time + 0.0001;
    time_count = time;
end
end

== matlab function nfo/Algorithm/Enabled Subsystem/IF Theta Switch  ==
  data: Time input; sensorless_theta output; IF_Theta input; Obe_Theta input; one input; zero input; Switch_time input; theta_compa output; switch_flag output
function [sensorless_theta,theta_compa,switch_flag] = fcn(Time,IF_Theta,Obe_Theta,one,zero,Switch_time)

sensorless_theta = zero;
theta_compa = zero;
switch_flag = zero;

%定义变量
persistent theta_give theta_comp last_error last_comp flag
if isempty(theta_give)
    theta_give = zero+0.2;
    theta_comp = zero;
    last_error = zero;
    last_comp = zero;
    flag = zero; %if角度切花obe角度的标志位
end

if(flag==1)
    sensorless_theta = Obe_Theta; %使用观测器角度
end


if(Time<Switch_time && flag==0)
    %还没到切换时间，并且切换标志位不成立，使用if角度
    sensorless_theta = IF_Theta;
elseif(Switch_time<=Time && Time<=Switch_time+0.05 && flag==0)
    %超过切换时间，并且低于切换时间+0.05，开始切换
    %惯性环节 1/(1+0.01s)
    theta_comp = 0.009950166250832*last_error + 0.990049833749168*last_comp; %???
    theta_compa = theta_comp;
    theta_give = IF_Theta + theta_comp;
    sensorless_theta = theta_give;

    if(sensorless_theta-Obe_Theta <0.1 && sensorless_theta-Obe_Theta>-0.1)
        flag = one;
    end
end

last_error = (Obe_Theta - IF_Theta);
last_comp = theta_comp;

if(sensorless_theta-Obe_Theta <0.2 && sensorless_theta-Obe_Theta>-0.2)
    switch_flag=one;
end
